simulink model "twin"  (R2018a)
settings: Solver=FixedStepAuto  StartTime=0.0  StopTime=3  FixedStep=0.01  RelTol=1e-3
values from neighbouring files (symbols this model uses):
  B = [-0.5     0       0.5     0 ... (first row only)    [DP_LPCA_based_prio.m]    (also in DPscaled_LPCA_based_prio.m; DPscaled_LPCA_based_prio_by_m1.m; SHC09.m = I \ [-l1, -l1*cos(d),  l1*cos(d),  l1,  l1*cos(d), -l1*cos(d; SHW09_vtol.m = zeros(3, 8))
  plim = [umin umax]    [derivative_DF.m]    (also in difference.m; quad.m; quad_tau.m; restoring_2d.m)
undefined symbols (not defined in the file or in its folder): a_c, a_t, Am, com_c, com_t_dca, com_t_inv, com_t_wls, p_limits, select_test, sigbuilder_block, v_limits
libraries: simulink x4, qcatlib x3, aerolibactuator x3
settings Model: Creator=mengc  LastModifiedBy=Ducted Fan

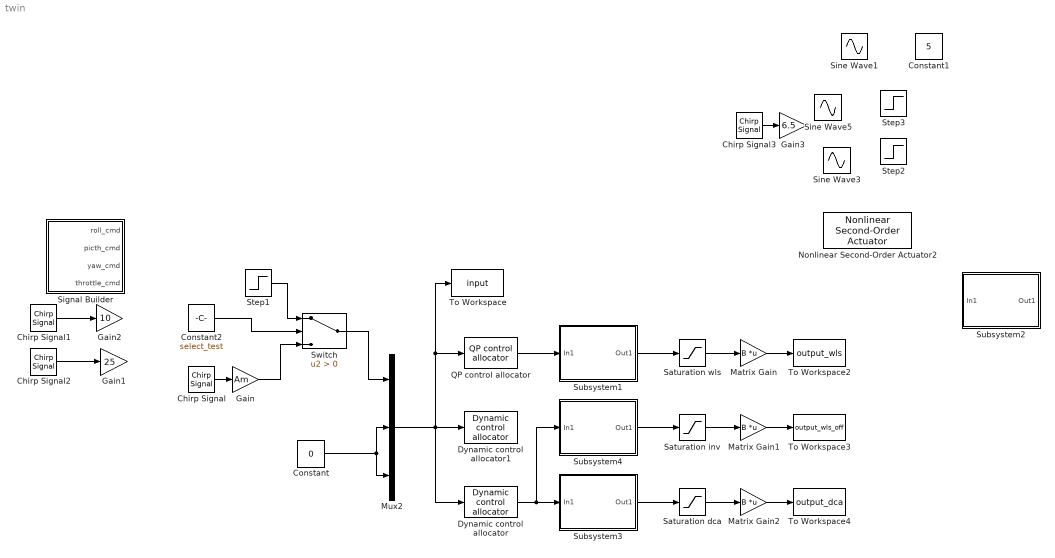
== system twin ==
  Chirp Signal : simulink/Sources/Chirp Signal  f1=lf  T=3  f2=hf
  Chirp Signal1 : simulink/Sources/Chirp Signal  f1=1  T=2  f2=5
  Chirp Signal2 : simulink/Sources/Chirp Signal  f1=1  T=2  f2=5
  Chirp Signal3 : simulink/Sources/Chirp Signal  f1=2  T=2  f2=6
  Constant : Constant  Value=0  SampleTime=0.01
  Constant1 : Constant  Value=5  SampleTime=0.01
  Constant2 : Constant  Value=select_test  SampleTime=0.01
  Dynamic control allocator : qcatlib/Dynamic control allocator  B=B  plim=plim  rlim=rlim  T=0.01  Wv=eye(3)  W1=dca_W1  W2=dca_W2  S=S
      settings: SourceProductName=QP Control Allocation Toolbox
  Dynamic control allocator1 : qcatlib/Dynamic control allocator  B=B  plim=plim  rlim=rlim  T=0.01  Wv=eye(3)  W1=eye(9)  W2=zeros(9,9)  S=S
      settings: SourceProductName=QP Control Allocation Toolbox
  Gain : Gain  Gain=Am
  Gain1 : Gain  Gain=25
  Gain2 : Gain  Gain=10
  Gain3 : Gain  Gain=6.5
  Matrix Gain : Gain  Gain=B  Multiplication=Matrix(K*u)  SaturateOnIntegerOverflow=on  OutDataTypeStr=Inherit: Same as input  ParamDataTypeStr=Inherit: Same as input
  Matrix Gain1 : Gain  Gain=B  Multiplication=Matrix(K*u)  SaturateOnIntegerOverflow=on  OutDataTypeStr=Inherit: Same as input  ParamDataTypeStr=Inherit: Same as input
  Matrix Gain2 : Gain  Gain=B  Multiplication=Matrix(K*u)  SaturateOnIntegerOverflow=on  OutDataTypeStr=Inherit: Same as input  ParamDataTypeStr=Inherit: Same as input
  Mux2 : Mux  Inputs=3
  Nonlinear Second-Order Actuator2 : aerolibactuator/Nonlinear Second-Order Actuator  wn_fin=200  z_fin=0.7  fin_max=umax  fin_min=umin  fin_maxrate=vmax  fin_act_0=zeros(9,1)  fin_act_vel=zeros(9,1)
      settings: SourceProductName=Aerospace Blockset  SourceProductBaseCode=AE
  QP control allocator : qcatlib/QP control allocator  B=B  plim=plim  rlim=rlim  T=0.01  Wv=eye(3)  Wu=eye(9)  ud=zeros(9,1)  alg=WLS  imax=100  gam=1e6  tol=1e-4
      settings: SourceProductName=QP Control Allocation Toolbox
  Saturation dca : Saturate  UpperLimit=plim(:,2)  LowerLimit=plim(:,1)
  Saturation inv : Saturate  UpperLimit=plim(:,2)  LowerLimit=plim(:,1)
  Saturation wls : Saturate  UpperLimit=plim(:,2)  LowerLimit=plim(:,1)
  Signal Builder : Subsystem  Tag=STV Subsys  LoadFcn=sigbuilder_block('load');  StartFcn=sigbuilder_block('start');  StopFcn=sigbuilder_block('stop');  ClipboardFcn=sigbuilder_block('clipboard');  mask(Sigbuilder block){tuvar=[0:10]}
      mask help: Simulink:masks:SigbuilderBlock_MD
      mask init:
      | if ~strcmp(get_param(bdroot(gcbh),'SimulationStatus'),'stopped') tuvar = sigbuilder_block('maskInit'); end
      settings: CopyFcn=sigbuilder_block('copy');  DeleteFcn=sigbuilder_block('delete');  ModelCloseFcn=sigbuilder_block('modelClose');  PreSaveFcn=sigbuilder_block('preSave');  PauseFcn=sigbuilder_block('pause');  ContinueFcn=sigbuilder_block('continue');  NameChangeFcn=sigbuilder_block('namechange');  OpenFcn=sigbuilder_block('open',[42.75 46.5 943.5 423.75 ]);  CloseFcn=sigbuilder_block('close');
      mask Display: plot(0, 0, 100, 100,[2, 2, 32, 32, 2], [68, 8, 8, 68, 68],[32, 2], [38, 38], [32, 19, 2],[53, 60, 44], [32, 17, 17, 2],[16, 16, 31, 31]);txt = getActiveGroup(gcbh);text(2, 100, txt,'verticalAlignment', 'top');
  Sine Wave1 : Sin  Amplitude=12  Frequency=4*pi/2  Phase=pi/2  SampleTime=0.01
  Sine Wave3 : Sin  Amplitude=15  Frequency=4*pi/2  Phase=pi/2  SampleTime=0.01
  Sine Wave5 : Sin  Amplitude=5  Frequency=4*pi/2  SampleTime=0.01
  Step1 : Step  Time=0.2  After=6  SampleTime=0.01
  Step2 : Step  Time=0.5  After=3  SampleTime=0.01
  Step3 : Step  Time=0.5  After=3  SampleTime=0.01
  Subsystem1 : Subsystem
  Subsystem2 : Subsystem
  Subsystem3 : Subsystem
  Subsystem4 : Subsystem
  Switch : Switch  Criteria=u2 > Threshold
  To Workspace : ToWorkspace  VariableName=input  SaveFormat=Timeseries  SampleTime=-1
  To Workspace2 : ToWorkspace  VariableName=output_wls  SaveFormat=Timeseries  SampleTime=-1
  To Workspace3 : ToWorkspace  VariableName=output_wls_off  SaveFormat=Timeseries  SampleTime=-1
  To Workspace4 : ToWorkspace  VariableName=output_dca  SaveFormat=Timeseries  SampleTime=-1
  wires:
  Mux2/1 -> Dynamic control allocator1/1, To Workspace/1, QP control allocator/1, Dynamic control allocator/1
  Matrix Gain/1 -> To Workspace2/1
  Matrix Gain2/1 -> To Workspace4/1
  Dynamic control allocator/1 -> Subsystem3/1(In1), Subsystem4/1(In1)
  Matrix Gain1/1 -> To Workspace3/1
  Subsystem3/1(Out1) -> Saturation dca/1
  Subsystem4/1(Out1) -> Saturation inv/1
  Subsystem1/1(Out1) -> Saturation wls/1
  QP control allocator/1 -> Subsystem1/1(In1)
  Saturation wls/1 -> Matrix Gain/1
  Saturation inv/1 -> Matrix Gain1/1
  Saturation dca/1 -> Matrix Gain2/1
  Chirp Signal2/1 -> Gain1/1
  Chirp Signal1/1 -> Gain2/1
  Chirp Signal/1 -> Gain/1
  Chirp Signal3/1 -> Gain3/1
  Constant/1 -> Mux2/3, Mux2/2
  Step1/1 -> Switch/1
  Gain/1 -> Switch/3
  Constant2/1 -> Switch/2
  Switch/1 -> Mux2/1

== system twin/Signal Builder ==
  Demux : Demux  Tag=STV Demux
  FromWs : FromWorkspace  Tag=STV FromWs  VariableName=tuvar  SampleTime=0
      SigBuilderData=|
      | common.afterFinalStr = 'Extrapolate'
      | common.sampleTime = 0
      | dataSet.timeRange = [0 100]
      | dataSet.name = 'Group 1'
      | sbobj.Groups.Name = 'Group 1'
      | sbobj.Groups.Signals(1).Name = 'roll_cmd'
      | sbobj.Groups.Signals(1).XData = [0 0.5 0.5 100]
      | sbobj.Groups.Signals(1).YData = [0 0 5 10]
      | sbobj.Groups.Signals(2).Name = 'picth_cmd'
      | sbobj.Groups.Signals(2).XData = [0 30 30 100]
      | sbobj.Groups.Signals(2).YData = [-0.0045 -0.0045 0.3 0.3]
      | sbobj.Groups.Signals(3).Name = 'yaw_cmd'
      | sbobj.Groups.Signals(3).XData = [0 30 30 100]
      | sbobj.Groups.Signals(3).YData = [0.0779 0.0779 0.2 0.2]
      | sbobj.Groups.Signals(4).Name = 'throttle_cmd'
      | sbobj.Groups.Signals(4).XData = [0 100]
      | sbobj.Groups.Signals(4).YData = [0 0]
      | sbobj.Groups.TimeRange = [0 100]
  roll_cmd : Outport  Tag=STV Outport
  picth_cmd : Outport  Tag=STV Outport  Port=2
  yaw_cmd : Outport  Tag=STV Outport  Port=3
  throttle_cmd : Outport  Tag=STV Outport  Port=4
  wires:
  Demux/1 -> roll_cmd/1
  FromWs/1 -> Demux/1
  Demux/2 -> picth_cmd/1
  Demux/3 -> yaw_cmd/1
  Demux/4 -> throttle_cmd/1

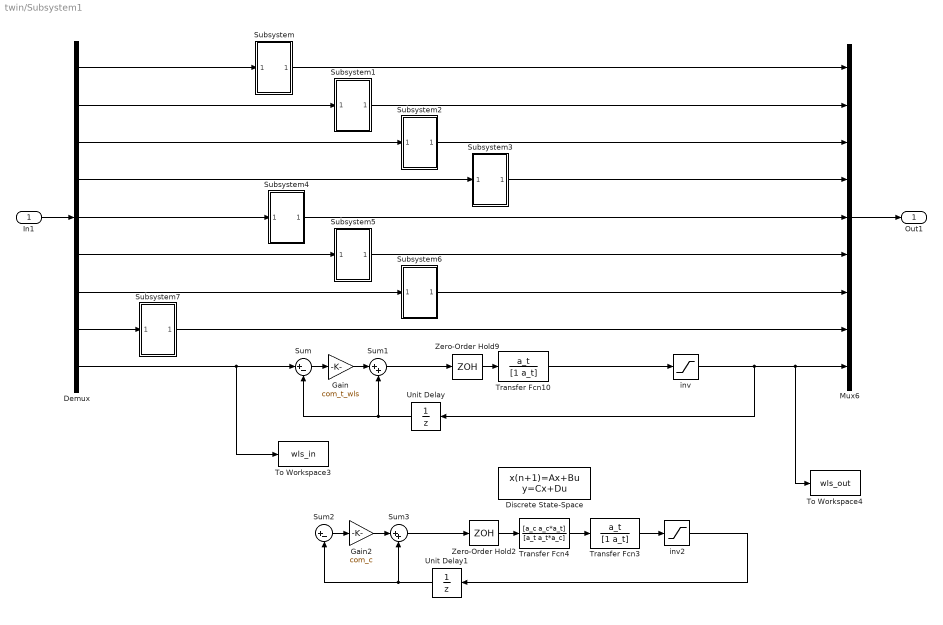
== system twin/Subsystem1 ==
  In1 : Inport
  Demux : Demux  Outputs=9
  Discrete State-Space : DiscreteStateSpace  A=exp(-0.01*a_t)  B=1-exp(-0.01*a_t)  D=0  SampleTime=-1
  Gain : Gain  Gain=com_t_wls
  Gain2 : Gain  Gain=com_c
  Mux6 : Mux  Inputs=9
  Subsystem : Subsystem
  Subsystem1 : Subsystem
  Subsystem2 : Subsystem
  Subsystem3 : Subsystem
  Subsystem4 : Subsystem
  Subsystem5 : Subsystem
  Subsystem6 : Subsystem
  Subsystem7 : Subsystem
  Sum : Sum  Inputs=|+-
  Sum1 : Sum  Inputs=|++
  Sum2 : Sum  Inputs=|+-
  Sum3 : Sum  Inputs=|++
  To Workspace3 : ToWorkspace  VariableName=wls_in  SaveFormat=Timeseries  SampleTime=-1
  To Workspace4 : ToWorkspace  VariableName=wls_out  SaveFormat=Timeseries  SampleTime=-1
  Transfer Fcn10 : TransferFcn  Numerator=a_t  Denominator=[1 a_t]
  Transfer Fcn3 : TransferFcn  Numerator=a_t  Denominator=[1 a_t]
  Transfer Fcn4 : TransferFcn  Numerator=[a_c a_c*a_t]  Denominator=[a_t a_t*a_c]
  Unit Delay : UnitDelay  SampleTime=-1
  Unit Delay1 : UnitDelay  SampleTime=-1
  Zero-Order Hold2 : ZeroOrderHold  SampleTime=-1
  Zero-Order Hold9 : ZeroOrderHold  SampleTime=-1
  inv : Saturate  UpperLimit=p_limits(2)  LowerLimit=-p_limits(2)
  inv2 : Saturate  UpperLimit=p_limits(2)  LowerLimit=-p_limits(2)
  Out1 : Outport
  wires:
  In1/1 -> Demux/1
  Mux6/1 -> Out1/1
  Gain/1 -> Sum1/1
  Zero-Order Hold9/1 -> Transfer Fcn10/1
  Unit Delay/1 -> Sum/2, Sum1/2
  Sum/1 -> Gain/1
  Sum1/1 -> Zero-Order Hold9/1
  Demux/1 -> Subsystem/1(In1)
  Subsystem/1(Out1) -> Mux6/1
  Demux/2 -> Subsystem1/1(In1)
  Subsystem1/1(Out1) -> Mux6/2
  Demux/3 -> Subsystem2/1(In1)
  Subsystem2/1(Out1) -> Mux6/3
  Demux/4 -> Subsystem3/1(In1)
  Subsystem3/1(Out1) -> Mux6/4
  Demux/5 -> Subsystem4/1(In1)
  Subsystem4/1(Out1) -> Mux6/5
  Demux/6 -> Subsystem5/1(In1)
  Subsystem5/1(Out1) -> Mux6/6
  Demux/7 -> Subsystem6/1(In1)
  Subsystem6/1(Out1) -> Mux6/7
  Subsystem7/1(Out1) -> Mux6/8
  Demux/8 -> Subsystem7/1(In1)
  inv/1 -> To Workspace4/1, Mux6/9, Unit Delay/1
  Gain2/1 -> Sum3/1
  Sum2/1 -> Gain2/1
  Unit Delay1/1 -> Sum2/2, Sum3/2
  Transfer Fcn4/1 -> Transfer Fcn3/1
  Transfer Fcn3/1 -> inv2/1
  Zero-Order Hold2/1 -> Transfer Fcn4/1
  inv2/1 -> Unit Delay1/1
  Sum3/1 -> Zero-Order Hold2/1
  Transfer Fcn10/1 -> inv/1
  Demux/9 -> To Workspace3/1, Sum/1

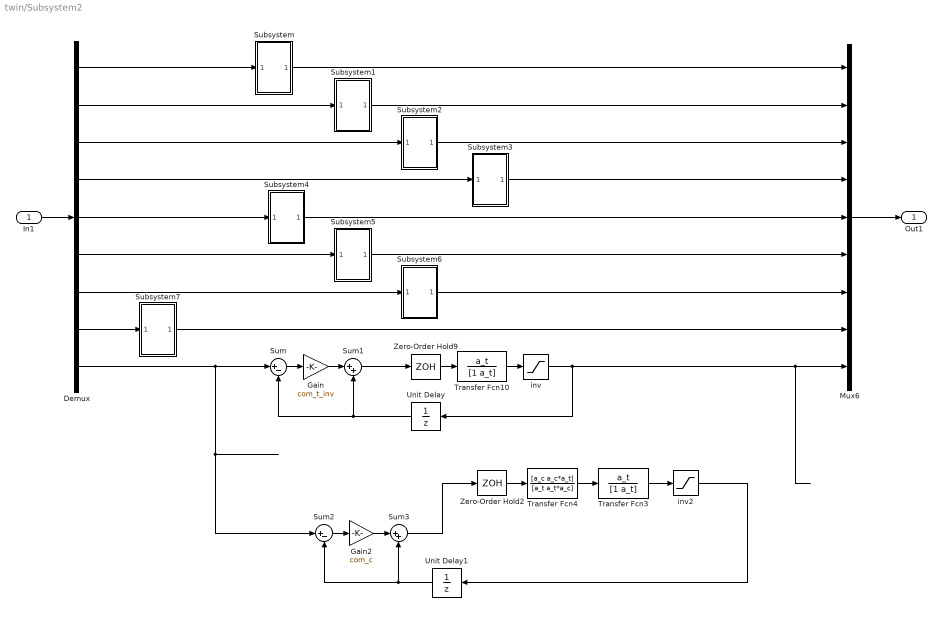
== system twin/Subsystem2 ==
  In1 : Inport
  Demux : Demux  Outputs=9
  Gain : Gain  Gain=com_t_inv
  Gain2 : Gain  Gain=com_c
  Mux6 : Mux  Inputs=9
  Subsystem : Subsystem
  Subsystem1 : Subsystem
  Subsystem2 : Subsystem
  Subsystem3 : Subsystem
  Subsystem4 : Subsystem
  Subsystem5 : Subsystem
  Subsystem6 : Subsystem
  Subsystem7 : Subsystem
  Sum : Sum  Inputs=|+-
  Sum1 : Sum  Inputs=|++
  Sum2 : Sum  Inputs=|+-
  Sum3 : Sum  Inputs=|++
  Transfer Fcn10 : TransferFcn  Numerator=a_t  Denominator=[1 a_t]
  Transfer Fcn3 : TransferFcn  Numerator=a_t  Denominator=[1 a_t]
  Transfer Fcn4 : TransferFcn  Numerator=[a_c a_c*a_t]  Denominator=[a_t a_t*a_c]
  Unit Delay : UnitDelay  SampleTime=-1
  Unit Delay1 : UnitDelay  SampleTime=-1
  Zero-Order Hold2 : ZeroOrderHold  SampleTime=-1
  Zero-Order Hold9 : ZeroOrderHold  SampleTime=-1
  inv : Saturate  UpperLimit=p_limits(2)  LowerLimit=-p_limits(2)
  inv2 : Saturate  UpperLimit=p_limits(2)  LowerLimit=-p_limits(2)
  Out1 : Outport
  wires:
  In1/1 -> Demux/1
  Mux6/1 -> Out1/1
  Transfer Fcn10/1 -> inv/1
  Gain/1 -> Sum1/1
  Zero-Order Hold9/1 -> Transfer Fcn10/1
  Unit Delay/1 -> Sum/2, Sum1/2
  Sum/1 -> Gain/1
  Demux/1 -> Subsystem/1(In1)
  Subsystem/1(Out1) -> Mux6/1
  Demux/2 -> Subsystem1/1(In1)
  Subsystem1/1(Out1) -> Mux6/2
  Demux/3 -> Subsystem2/1(In1)
  Subsystem2/1(Out1) -> Mux6/3
  Demux/4 -> Subsystem3/1(In1)
  Subsystem3/1(Out1) -> Mux6/4
  Demux/5 -> Subsystem4/1(In1)
  Subsystem4/1(Out1) -> Mux6/5
  Demux/6 -> Subsystem5/1(In1)
  Subsystem5/1(Out1) -> Mux6/6
  Demux/7 -> Subsystem6/1(In1)
  Subsystem6/1(Out1) -> Mux6/7
  Subsystem7/1(Out1) -> Mux6/8
  Demux/8 -> Subsystem7/1(In1)
  inv/1 -> Mux6/9, Unit Delay/1
  Gain2/1 -> Sum3/1
  Sum2/1 -> Gain2/1
  Unit Delay1/1 -> Sum2/2, Sum3/2
  Transfer Fcn4/1 -> Transfer Fcn3/1
  Transfer Fcn3/1 -> inv2/1
  Zero-Order Hold2/1 -> Transfer Fcn4/1
  inv2/1 -> Unit Delay1/1
  Sum3/1 -> Zero-Order Hold2/1
  Demux/9 -> Sum/1, Sum2/1
  Sum1/1 -> Zero-Order Hold9/1

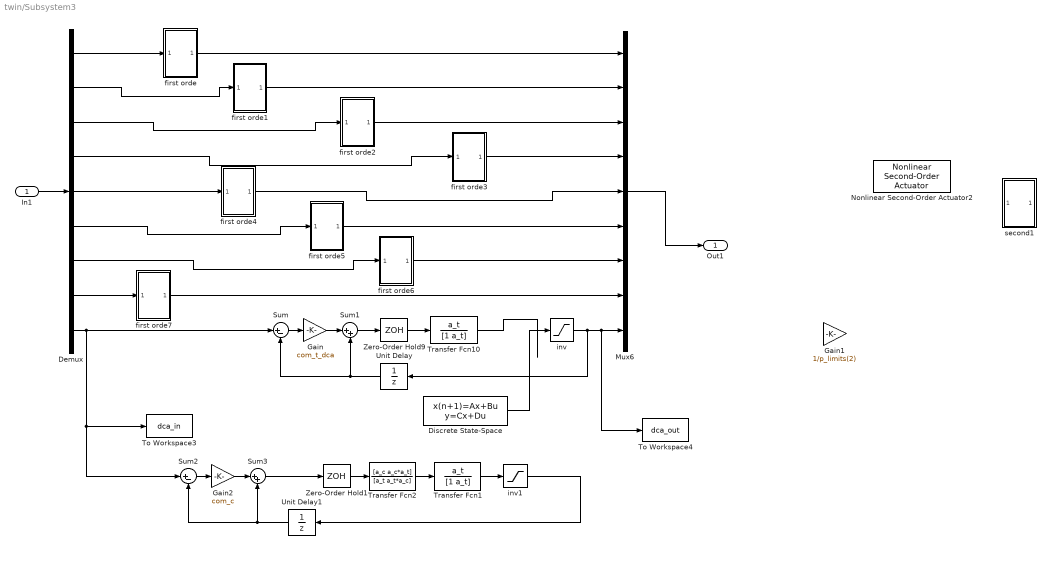
== system twin/Subsystem3 ==
  In1 : Inport
  Demux : Demux  Outputs=9
  Discrete State-Space : DiscreteStateSpace  A=exp(-0.01*a_t)  B=1-exp(-0.01*a_t)  D=0  SampleTime=-1
  Gain : Gain  Gain=com_t_dca
  Gain1 : Gain  Gain=1/p_limits(2)
  Gain2 : Gain  Gain=com_c
  Mux6 : Mux  Inputs=9
  Nonlinear Second-Order Actuator2 : aerolibactuator/Nonlinear Second-Order Actuator  wn_fin=200  z_fin=0.7  fin_max=(p_limits(2))*pi/180  fin_min=(-p_limits(2))*pi/180  fin_maxrate=v_limits(2)  fin_act_0=0  fin_act_vel=0
      settings: SourceProductName=Aerospace Blockset  SourceProductBaseCode=AE
  Sum : Sum  Inputs=|+-
  Sum1 : Sum  Inputs=|++
  Sum2 : Sum  Inputs=|+-
  Sum3 : Sum  Inputs=|++
  To Workspace3 : ToWorkspace  VariableName=dca_in  SaveFormat=Timeseries  SampleTime=-1
  To Workspace4 : ToWorkspace  VariableName=dca_out  SaveFormat=Timeseries  SampleTime=-1
  Transfer Fcn1 : TransferFcn  Numerator=a_t  Denominator=[1 a_t]
  Transfer Fcn10 : TransferFcn  Numerator=a_t  Denominator=[1 a_t]
  Transfer Fcn2 : TransferFcn  Numerator=[a_c a_c*a_t]  Denominator=[a_t a_t*a_c]
  Unit Delay : UnitDelay  SampleTime=-1
  Unit Delay1 : UnitDelay  SampleTime=-1
  Zero-Order Hold1 : ZeroOrderHold  SampleTime=-1
  Zero-Order Hold9 : ZeroOrderHold  SampleTime=-1
  first orde : Subsystem
  first orde1 : Subsystem
  first orde2 : Subsystem
  first orde3 : Subsystem
  first orde4 : Subsystem
  first orde5 : Subsystem
  first orde6 : Subsystem
  first orde7 : Subsystem
  inv : Saturate  UpperLimit=p_limits(2)  LowerLimit=-p_limits(2)
  inv1 : Saturate  UpperLimit=p_limits(2)  LowerLimit=-p_limits(2)
  second1 : Subsystem
  Out1 : Outport
  wires:
  In1/1 -> Demux/1
  Mux6/1 -> Out1/1
  Gain/1 -> Sum1/1
  Unit Delay/1 -> Sum/2, Sum1/2
  Sum/1 -> Gain/1
  Sum1/1 -> Zero-Order Hold9/1
  Demux/1 -> first orde/1(In1)
  first orde/1(Out1) -> Mux6/1
  Demux/2 -> first orde1/1(In1)
  first orde1/1(Out1) -> Mux6/2
  Demux/3 -> first orde2/1(In1)
  first orde2/1(Out1) -> Mux6/3
  Demux/4 -> first orde3/1(In1)
  first orde3/1(Out1) -> Mux6/4
  Demux/5 -> first orde4/1(In1)
  first orde4/1(Out1) -> Mux6/5
  Demux/6 -> first orde5/1(In1)
  first orde5/1(Out1) -> Mux6/6
  Demux/7 -> first orde6/1(In1)
  first orde6/1(Out1) -> Mux6/7
  first orde7/1(Out1) -> Mux6/8
  Demux/8 -> first orde7/1(In1)
  Transfer Fcn10/1 -> inv/1
  inv/1 -> To Workspace4/1, Mux6/9, Unit Delay/1
  Transfer Fcn1/1 -> inv1/1
  Zero-Order Hold1/1 -> Transfer Fcn2/1
  Transfer Fcn2/1 -> Transfer Fcn1/1
  inv1/1 -> Unit Delay1/1
  Sum3/1 -> Zero-Order Hold1/1
  Unit Delay1/1 -> Sum2/2, Sum3/2
  Sum2/1 -> Gain2/1
  Gain2/1 -> Sum3/1
  Demux/9 -> Sum2/1, To Workspace3/1, Sum/1
  Discrete State-Space/1 -> ?
  Zero-Order Hold9/1 -> Transfer Fcn10/1

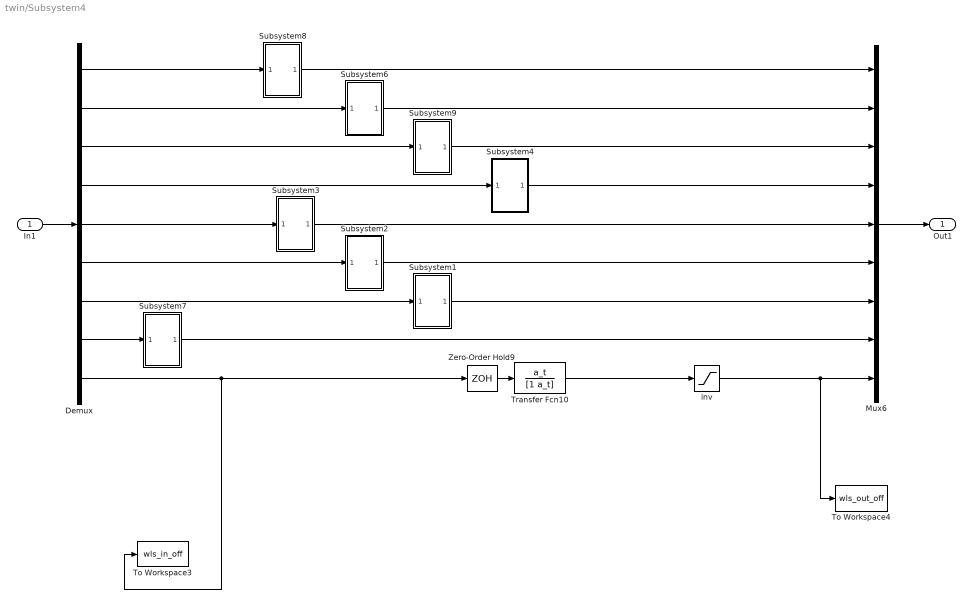
== system twin/Subsystem4 ==
  In1 : Inport
  Demux : Demux  Outputs=9
  Mux6 : Mux  Inputs=9
  Subsystem1 : Subsystem
  Subsystem2 : Subsystem
  Subsystem3 : Subsystem
  Subsystem4 : Subsystem
  Subsystem6 : Subsystem
  Subsystem7 : Subsystem
  Subsystem8 : Subsystem
  Subsystem9 : Subsystem
  To Workspace3 : ToWorkspace  VariableName=wls_in_off  SaveFormat=Timeseries  SampleTime=-1
  To Workspace4 : ToWorkspace  VariableName=wls_out_off  SaveFormat=Timeseries  SampleTime=-1
  Transfer Fcn10 : TransferFcn  Numerator=a_t  Denominator=[1 a_t]
  Zero-Order Hold9 : ZeroOrderHold  SampleTime=-1
  inv : Saturate  UpperLimit=p_limits(2)  LowerLimit=-p_limits(2)
  Out1 : Outport
  wires:
  In1/1 -> Demux/1
  Mux6/1 -> Out1/1
  Zero-Order Hold9/1 -> Transfer Fcn10/1
  Demux/1 -> Subsystem8/1(In1)
  Subsystem8/1(Out1) -> Mux6/1
  Demux/2 -> Subsystem6/1(In1)
  Subsystem6/1(Out1) -> Mux6/2
  Demux/3 -> Subsystem9/1(In1)
  Subsystem9/1(Out1) -> Mux6/3
  Demux/4 -> Subsystem4/1(In1)
  Subsystem4/1(Out1) -> Mux6/4
  Demux/5 -> Subsystem3/1(In1)
  Subsystem3/1(Out1) -> Mux6/5
  Demux/6 -> Subsystem2/1(In1)
  Subsystem2/1(Out1) -> Mux6/6
  Demux/7 -> Subsystem1/1(In1)
  Subsystem1/1(Out1) -> Mux6/7
  Subsystem7/1(Out1) -> Mux6/8
  Demux/8 -> Subsystem7/1(In1)
  inv/1 -> To Workspace4/1, Mux6/9
  Demux/9 -> Zero-Order Hold9/1, To Workspace3/1
  Transfer Fcn10/1 -> inv/1

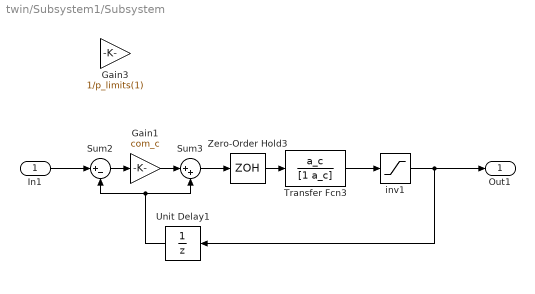
== system twin/Subsystem1/Subsystem ==
  In1 : Inport
  Gain1 : Gain  Gain=com_c
  Gain3 : Gain  Gain=1/p_limits(1)
  Sum2 : Sum  Inputs=|+-
  Sum3 : Sum  Inputs=|++
  Transfer Fcn3 : TransferFcn  Numerator=a_c  Denominator=[1 a_c]
  Unit Delay1 : UnitDelay  SampleTime=-1
  Zero-Order Hold3 : ZeroOrderHold  SampleTime=-1
  inv1 : Saturate  UpperLimit=p_limits(1)  LowerLimit=-p_limits(1)
  Out1 : Outport
  wires:
  Transfer Fcn3/1 -> inv1/1
  Gain1/1 -> Sum3/1
  Unit Delay1/1 -> Sum2/2, Sum3/2
  Sum2/1 -> Gain1/1
  Zero-Order Hold3/1 -> Transfer Fcn3/1
  Sum3/1 -> Zero-Order Hold3/1
  inv1/1 -> Unit Delay1/1, Out1/1
  In1/1 -> Sum2/1

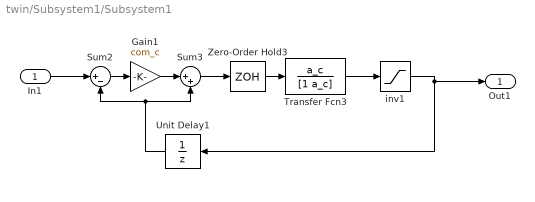
== system twin/Subsystem1/Subsystem1 ==
  In1 : Inport
  Gain1 : Gain  Gain=com_c
  Sum2 : Sum  Inputs=|+-
  Sum3 : Sum  Inputs=|++
  Transfer Fcn3 : TransferFcn  Numerator=a_c  Denominator=[1 a_c]
  Unit Delay1 : UnitDelay  SampleTime=-1
  Zero-Order Hold3 : ZeroOrderHold  SampleTime=-1
  inv1 : Saturate  UpperLimit=p_limits(1)  LowerLimit=-p_limits(1)
  Out1 : Outport
  wires:
  Transfer Fcn3/1 -> inv1/1
  Gain1/1 -> Sum3/1
  inv1/1 -> Unit Delay1/1, Out1/1
  In1/1 -> Sum2/1
  Unit Delay1/1 -> Sum2/2, Sum3/2
  Sum2/1 -> Gain1/1
  Zero-Order Hold3/1 -> Transfer Fcn3/1
  Sum3/1 -> Zero-Order Hold3/1

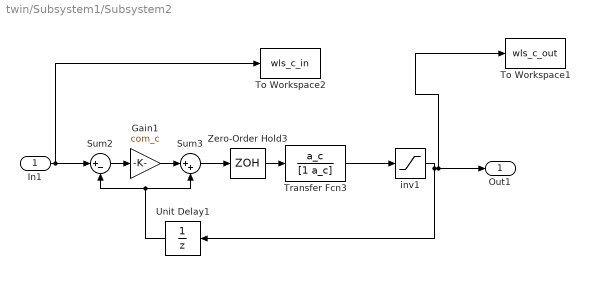
== system twin/Subsystem1/Subsystem2 ==
  In1 : Inport
  Gain1 : Gain  Gain=com_c
  Sum2 : Sum  Inputs=|+-
  Sum3 : Sum  Inputs=|++
  To Workspace1 : ToWorkspace  VariableName=wls_c_out  SaveFormat=Timeseries  SampleTime=-1
  To Workspace2 : ToWorkspace  VariableName=wls_c_in  SaveFormat=Timeseries  SampleTime=-1
  Transfer Fcn3 : TransferFcn  Numerator=a_c  Denominator=[1 a_c]
  Unit Delay1 : UnitDelay  SampleTime=-1
  Zero-Order Hold3 : ZeroOrderHold  SampleTime=-1
  inv1 : Saturate  UpperLimit=p_limits(1)  LowerLimit=-p_limits(1)
  Out1 : Outport
  wires:
  Gain1/1 -> Sum3/1
  Unit Delay1/1 -> Sum2/2, Sum3/2
  Sum2/1 -> Gain1/1
  Zero-Order Hold3/1 -> Transfer Fcn3/1
  Sum3/1 -> Zero-Order Hold3/1
  In1/1 -> To Workspace2/1, Sum2/1
  inv1/1 -> Unit Delay1/1, To Workspace1/1, Out1/1
  Transfer Fcn3/1 -> inv1/1

== system twin/Subsystem1/Subsystem3 ==
  In1 : Inport
  Gain1 : Gain  Gain=com_c
  Sum2 : Sum  Inputs=|+-
  Sum3 : Sum  Inputs=|++
  Transfer Fcn3 : TransferFcn  Numerator=a_c  Denominator=[1 a_c]
  Unit Delay1 : UnitDelay  SampleTime=-1
  Zero-Order Hold3 : ZeroOrderHold  SampleTime=-1
  inv1 : Saturate  UpperLimit=p_limits(1)  LowerLimit=-p_limits(1)
  Out1 : Outport
  wires:
  Transfer Fcn3/1 -> inv1/1
  Gain1/1 -> Sum3/1
  inv1/1 -> Unit Delay1/1, Out1/1
  In1/1 -> Sum2/1
  Unit Delay1/1 -> Sum2/2, Sum3/2
  Sum2/1 -> Gain1/1
  Zero-Order Hold3/1 -> Transfer Fcn3/1
  Sum3/1 -> Zero-Order Hold3/1

== system twin/Subsystem1/Subsystem4 ==
  In1 : Inport
  Gain1 : Gain  Gain=com_c
  Sum2 : Sum  Inputs=|+-
  Sum3 : Sum  Inputs=|++
  Transfer Fcn3 : TransferFcn  Numerator=a_c  Denominator=[1 a_c]
  Unit Delay1 : UnitDelay  SampleTime=-1
  Zero-Order Hold3 : ZeroOrderHold  SampleTime=-1
  inv1 : Saturate  UpperLimit=p_limits(1)  LowerLimit=-p_limits(1)
  Out1 : Outport
  wires:
  Transfer Fcn3/1 -> inv1/1
  Gain1/1 -> Sum3/1
  inv1/1 -> Unit Delay1/1, Out1/1
  In1/1 -> Sum2/1
  Unit Delay1/1 -> Sum2/2, Sum3/2
  Sum2/1 -> Gain1/1
  Zero-Order Hold3/1 -> Transfer Fcn3/1
  Sum3/1 -> Zero-Order Hold3/1

== system twin/Subsystem1/Subsystem5 ==
  In1 : Inport
  Gain1 : Gain  Gain=com_c
  Sum2 : Sum  Inputs=|+-
  Sum3 : Sum  Inputs=|++
  Transfer Fcn3 : TransferFcn  Numerator=a_c  Denominator=[1 a_c]
  Unit Delay1 : UnitDelay  SampleTime=-1
  Zero-Order Hold3 : ZeroOrderHold  SampleTime=-1
  inv1 : Saturate  UpperLimit=p_limits(1)  LowerLimit=-p_limits(1)
  Out1 : Outport
  wires:
  Transfer Fcn3/1 -> inv1/1
  Gain1/1 -> Sum3/1
  inv1/1 -> Unit Delay1/1, Out1/1
  In1/1 -> Sum2/1
  Unit Delay1/1 -> Sum2/2, Sum3/2
  Sum2/1 -> Gain1/1
  Zero-Order Hold3/1 -> Transfer Fcn3/1
  Sum3/1 -> Zero-Order Hold3/1

== system twin/Subsystem1/Subsystem6 ==
  In1 : Inport
  Gain1 : Gain  Gain=com_c
  Sum2 : Sum  Inputs=|+-
  Sum3 : Sum  Inputs=|++
  Transfer Fcn3 : TransferFcn  Numerator=a_c  Denominator=[1 a_c]
  Unit Delay1 : UnitDelay  SampleTime=-1
  Zero-Order Hold3 : ZeroOrderHold  SampleTime=-1
  inv1 : Saturate  UpperLimit=p_limits(1)  LowerLimit=-p_limits(1)
  Out1 : Outport
  wires:
  Transfer Fcn3/1 -> inv1/1
  Gain1/1 -> Sum3/1
  inv1/1 -> Unit Delay1/1, Out1/1
  In1/1 -> Sum2/1
  Unit Delay1/1 -> Sum2/2, Sum3/2
  Sum2/1 -> Gain1/1
  Zero-Order Hold3/1 -> Transfer Fcn3/1
  Sum3/1 -> Zero-Order Hold3/1

== system twin/Subsystem1/Subsystem7 ==
  In1 : Inport
  Gain1 : Gain  Gain=com_c
  Sum2 : Sum  Inputs=|+-
  Sum3 : Sum  Inputs=|++
  Transfer Fcn3 : TransferFcn  Numerator=a_c  Denominator=[1 a_c]
  Unit Delay1 : UnitDelay  SampleTime=-1
  Zero-Order Hold3 : ZeroOrderHold  SampleTime=-1
  inv1 : Saturate  UpperLimit=p_limits(1)  LowerLimit=-p_limits(1)
  Out1 : Outport
  wires:
  Transfer Fcn3/1 -> inv1/1
  Gain1/1 -> Sum3/1
  inv1/1 -> Unit Delay1/1, Out1/1
  In1/1 -> Sum2/1
  Unit Delay1/1 -> Sum2/2, Sum3/2
  Sum2/1 -> Gain1/1
  Zero-Order Hold3/1 -> Transfer Fcn3/1
  Sum3/1 -> Zero-Order Hold3/1

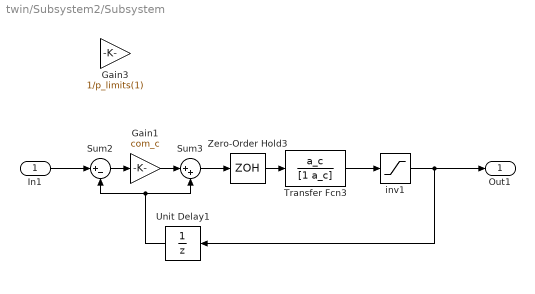
== system twin/Subsystem2/Subsystem ==
  In1 : Inport
  Gain1 : Gain  Gain=com_c
  Gain3 : Gain  Gain=1/p_limits(1)
  Sum2 : Sum  Inputs=|+-
  Sum3 : Sum  Inputs=|++
  Transfer Fcn3 : TransferFcn  Numerator=a_c  Denominator=[1 a_c]
  Unit Delay1 : UnitDelay  SampleTime=-1
  Zero-Order Hold3 : ZeroOrderHold  SampleTime=-1
  inv1 : Saturate  UpperLimit=p_limits(1)  LowerLimit=-p_limits(1)
  Out1 : Outport
  wires:
  Transfer Fcn3/1 -> inv1/1
  Gain1/1 -> Sum3/1
  Unit Delay1/1 -> Sum2/2, Sum3/2
  Sum2/1 -> Gain1/1
  Zero-Order Hold3/1 -> Transfer Fcn3/1
  Sum3/1 -> Zero-Order Hold3/1
  inv1/1 -> Unit Delay1/1, Out1/1
  In1/1 -> Sum2/1

== system twin/Subsystem2/Subsystem1 ==
  In1 : Inport
  Gain1 : Gain  Gain=com_c
  Sum2 : Sum  Inputs=|+-
  Sum3 : Sum  Inputs=|++
  Transfer Fcn3 : TransferFcn  Numerator=a_c  Denominator=[1 a_c]
  Unit Delay1 : UnitDelay  SampleTime=-1
  Zero-Order Hold3 : ZeroOrderHold  SampleTime=-1
  inv1 : Saturate  UpperLimit=p_limits(1)  LowerLimit=-p_limits(1)
  Out1 : Outport
  wires:
  Transfer Fcn3/1 -> inv1/1
  Gain1/1 -> Sum3/1
  inv1/1 -> Unit Delay1/1, Out1/1
  In1/1 -> Sum2/1
  Unit Delay1/1 -> Sum2/2, Sum3/2
  Sum2/1 -> Gain1/1
  Zero-Order Hold3/1 -> Transfer Fcn3/1
  Sum3/1 -> Zero-Order Hold3/1

== system twin/Subsystem2/Subsystem2 ==
  In1 : Inport
  Gain1 : Gain  Gain=com_c
  Sum2 : Sum  Inputs=|+-
  Sum3 : Sum  Inputs=|++
  Transfer Fcn3 : TransferFcn  Numerator=a_c  Denominator=[1 a_c]
  Unit Delay1 : UnitDelay  SampleTime=-1
  Zero-Order Hold3 : ZeroOrderHold  SampleTime=-1
  inv1 : Saturate  UpperLimit=p_limits(1)  LowerLimit=-p_limits(1)
  Out1 : Outport
  wires:
  Transfer Fcn3/1 -> inv1/1
  Gain1/1 -> Sum3/1
  inv1/1 -> Unit Delay1/1, Out1/1
  In1/1 -> Sum2/1
  Unit Delay1/1 -> Sum2/2, Sum3/2
  Sum2/1 -> Gain1/1
  Zero-Order Hold3/1 -> Transfer Fcn3/1
  Sum3/1 -> Zero-Order Hold3/1

== system twin/Subsystem2/Subsystem3 ==
  In1 : Inport
  Gain1 : Gain  Gain=com_c
  Sum2 : Sum  Inputs=|+-
  Sum3 : Sum  Inputs=|++
  Transfer Fcn3 : TransferFcn  Numerator=a_c  Denominator=[1 a_c]
  Unit Delay1 : UnitDelay  SampleTime=-1
  Zero-Order Hold3 : ZeroOrderHold  SampleTime=-1
  inv1 : Saturate  UpperLimit=p_limits(1)  LowerLimit=-p_limits(1)
  Out1 : Outport
  wires:
  Transfer Fcn3/1 -> inv1/1
  Gain1/1 -> Sum3/1
  inv1/1 -> Unit Delay1/1, Out1/1
  In1/1 -> Sum2/1
  Unit Delay1/1 -> Sum2/2, Sum3/2
  Sum2/1 -> Gain1/1
  Zero-Order Hold3/1 -> Transfer Fcn3/1
  Sum3/1 -> Zero-Order Hold3/1

== system twin/Subsystem2/Subsystem4 ==
  In1 : Inport
  Gain1 : Gain  Gain=com_c
  Sum2 : Sum  Inputs=|+-
  Sum3 : Sum  Inputs=|++
  Transfer Fcn3 : TransferFcn  Numerator=a_c  Denominator=[1 a_c]
  Unit Delay1 : UnitDelay  SampleTime=-1
  Zero-Order Hold3 : ZeroOrderHold  SampleTime=-1
  inv1 : Saturate  UpperLimit=p_limits(1)  LowerLimit=-p_limits(1)
  Out1 : Outport
  wires:
  Transfer Fcn3/1 -> inv1/1
  Gain1/1 -> Sum3/1
  inv1/1 -> Unit Delay1/1, Out1/1
  In1/1 -> Sum2/1
  Unit Delay1/1 -> Sum2/2, Sum3/2
  Sum2/1 -> Gain1/1
  Zero-Order Hold3/1 -> Transfer Fcn3/1
  Sum3/1 -> Zero-Order Hold3/1

== system twin/Subsystem2/Subsystem5 ==
  In1 : Inport
  Gain1 : Gain  Gain=com_c
  Sum2 : Sum  Inputs=|+-
  Sum3 : Sum  Inputs=|++
  Transfer Fcn3 : TransferFcn  Numerator=a_c  Denominator=[1 a_c]
  Unit Delay1 : UnitDelay  SampleTime=-1
  Zero-Order Hold3 : ZeroOrderHold  SampleTime=-1
  inv1 : Saturate  UpperLimit=p_limits(1)  LowerLimit=-p_limits(1)
  Out1 : Outport
  wires:
  Transfer Fcn3/1 -> inv1/1
  Gain1/1 -> Sum3/1
  inv1/1 -> Unit Delay1/1, Out1/1
  In1/1 -> Sum2/1
  Unit Delay1/1 -> Sum2/2, Sum3/2
  Sum2/1 -> Gain1/1
  Zero-Order Hold3/1 -> Transfer Fcn3/1
  Sum3/1 -> Zero-Order Hold3/1

== system twin/Subsystem2/Subsystem6 ==
  In1 : Inport
  Gain1 : Gain  Gain=com_c
  Sum2 : Sum  Inputs=|+-
  Sum3 : Sum  Inputs=|++
  Transfer Fcn3 : TransferFcn  Numerator=a_c  Denominator=[1 a_c]
  Unit Delay1 : UnitDelay  SampleTime=-1
  Zero-Order Hold3 : ZeroOrderHold  SampleTime=-1
  inv1 : Saturate  UpperLimit=p_limits(1)  LowerLimit=-p_limits(1)
  Out1 : Outport
  wires:
  Transfer Fcn3/1 -> inv1/1
  Gain1/1 -> Sum3/1
  inv1/1 -> Unit Delay1/1, Out1/1
  In1/1 -> Sum2/1
  Unit Delay1/1 -> Sum2/2, Sum3/2
  Sum2/1 -> Gain1/1
  Zero-Order Hold3/1 -> Transfer Fcn3/1
  Sum3/1 -> Zero-Order Hold3/1

== system twin/Subsystem2/Subsystem7 ==
  In1 : Inport
  Gain1 : Gain  Gain=com_c
  Sum2 : Sum  Inputs=|+-
  Sum3 : Sum  Inputs=|++
  Transfer Fcn3 : TransferFcn  Numerator=a_c  Denominator=[1 a_c]
  Unit Delay1 : UnitDelay  SampleTime=-1
  Zero-Order Hold3 : ZeroOrderHold  SampleTime=-1
  inv1 : Saturate  UpperLimit=p_limits(1)  LowerLimit=-p_limits(1)
  Out1 : Outport
  wires:
  Transfer Fcn3/1 -> inv1/1
  Gain1/1 -> Sum3/1
  inv1/1 -> Unit Delay1/1, Out1/1
  In1/1 -> Sum2/1
  Unit Delay1/1 -> Sum2/2, Sum3/2
  Sum2/1 -> Gain1/1
  Zero-Order Hold3/1 -> Transfer Fcn3/1
  Sum3/1 -> Zero-Order Hold3/1

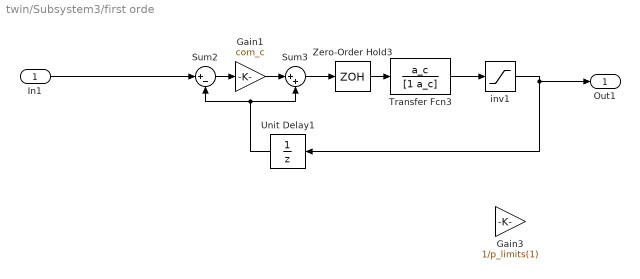
== system twin/Subsystem3/first orde ==
  In1 : Inport
  Gain1 : Gain  Gain=com_c
  Gain3 : Gain  Gain=1/p_limits(1)
  Sum2 : Sum  Inputs=|+-
  Sum3 : Sum  Inputs=|++
  Transfer Fcn3 : TransferFcn  Numerator=a_c  Denominator=[1 a_c]
  Unit Delay1 : UnitDelay  SampleTime=-1
  Zero-Order Hold3 : ZeroOrderHold  SampleTime=-1
  inv1 : Saturate  UpperLimit=p_limits(1)  LowerLimit=-p_limits(1)
  Out1 : Outport
  wires:
  Transfer Fcn3/1 -> inv1/1
  Gain1/1 -> Sum3/1
  Unit Delay1/1 -> Sum2/2, Sum3/2
  Sum2/1 -> Gain1/1
  Zero-Order Hold3/1 -> Transfer Fcn3/1
  Sum3/1 -> Zero-Order Hold3/1
  In1/1 -> Sum2/1
  inv1/1 -> Unit Delay1/1, Out1/1

== system twin/Subsystem3/first orde1 ==
  In1 : Inport
  Gain1 : Gain  Gain=com_c
  Sum2 : Sum  Inputs=|+-
  Sum3 : Sum  Inputs=|++
  Transfer Fcn3 : TransferFcn  Numerator=a_c  Denominator=[1 a_c]
  Unit Delay1 : UnitDelay  SampleTime=-1
  Zero-Order Hold3 : ZeroOrderHold  SampleTime=-1
  inv1 : Saturate  UpperLimit=p_limits(1)  LowerLimit=-p_limits(1)
  Out1 : Outport
  wires:
  Transfer Fcn3/1 -> inv1/1
  Gain1/1 -> Sum3/1
  inv1/1 -> Unit Delay1/1, Out1/1
  In1/1 -> Sum2/1
  Unit Delay1/1 -> Sum2/2, Sum3/2
  Sum2/1 -> Gain1/1
  Zero-Order Hold3/1 -> Transfer Fcn3/1
  Sum3/1 -> Zero-Order Hold3/1

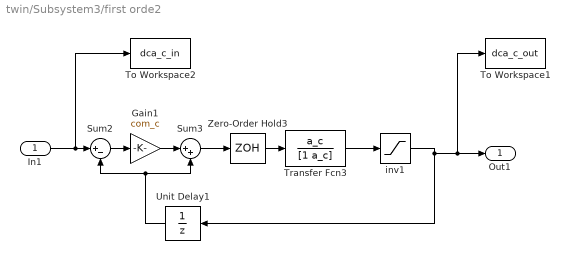
== system twin/Subsystem3/first orde2 ==
  In1 : Inport
  Gain1 : Gain  Gain=com_c
  Sum2 : Sum  Inputs=|+-
  Sum3 : Sum  Inputs=|++
  To Workspace1 : ToWorkspace  VariableName=dca_c_out  SaveFormat=Timeseries  SampleTime=-1
  To Workspace2 : ToWorkspace  VariableName=dca_c_in  SaveFormat=Timeseries  SampleTime=-1
  Transfer Fcn3 : TransferFcn  Numerator=a_c  Denominator=[1 a_c]
  Unit Delay1 : UnitDelay  SampleTime=-1
  Zero-Order Hold3 : ZeroOrderHold  SampleTime=-1
  inv1 : Saturate  UpperLimit=p_limits(1)  LowerLimit=-p_limits(1)
  Out1 : Outport
  wires:
  Transfer Fcn3/1 -> inv1/1
  Gain1/1 -> Sum3/1
  Unit Delay1/1 -> Sum2/2, Sum3/2
  Sum2/1 -> Gain1/1
  Zero-Order Hold3/1 -> Transfer Fcn3/1
  Sum3/1 -> Zero-Order Hold3/1
  inv1/1 -> Unit Delay1/1, To Workspace1/1, Out1/1
  In1/1 -> To Workspace2/1, Sum2/1

== system twin/Subsystem3/first orde3 ==
  In1 : Inport
  Gain1 : Gain  Gain=com_c
  Sum2 : Sum  Inputs=|+-
  Sum3 : Sum  Inputs=|++
  Transfer Fcn3 : TransferFcn  Numerator=a_c  Denominator=[1 a_c]
  Unit Delay1 : UnitDelay  SampleTime=-1
  Zero-Order Hold3 : ZeroOrderHold  SampleTime=-1
  inv1 : Saturate  UpperLimit=p_limits(1)  LowerLimit=-p_limits(1)
  Out1 : Outport
  wires:
  Transfer Fcn3/1 -> inv1/1
  Gain1/1 -> Sum3/1
  inv1/1 -> Unit Delay1/1, Out1/1
  In1/1 -> Sum2/1
  Unit Delay1/1 -> Sum2/2, Sum3/2
  Sum2/1 -> Gain1/1
  Zero-Order Hold3/1 -> Transfer Fcn3/1
  Sum3/1 -> Zero-Order Hold3/1

== system twin/Subsystem3/first orde4 ==
  In1 : Inport
  Gain1 : Gain  Gain=com_c
  Sum2 : Sum  Inputs=|+-
  Sum3 : Sum  Inputs=|++
  Transfer Fcn3 : TransferFcn  Numerator=a_c  Denominator=[1 a_c]
  Unit Delay1 : UnitDelay  SampleTime=-1
  Zero-Order Hold3 : ZeroOrderHold  SampleTime=-1
  inv1 : Saturate  UpperLimit=p_limits(1)  LowerLimit=-p_limits(1)
  Out1 : Outport
  wires:
  Transfer Fcn3/1 -> inv1/1
  Gain1/1 -> Sum3/1
  inv1/1 -> Unit Delay1/1, Out1/1
  In1/1 -> Sum2/1
  Unit Delay1/1 -> Sum2/2, Sum3/2
  Sum2/1 -> Gain1/1
  Zero-Order Hold3/1 -> Transfer Fcn3/1
  Sum3/1 -> Zero-Order Hold3/1

== system twin/Subsystem3/first orde5 ==
  In1 : Inport
  Gain1 : Gain  Gain=com_c
  Sum2 : Sum  Inputs=|+-
  Sum3 : Sum  Inputs=|++
  Transfer Fcn3 : TransferFcn  Numerator=a_c  Denominator=[1 a_c]
  Unit Delay1 : UnitDelay  SampleTime=-1
  Zero-Order Hold3 : ZeroOrderHold  SampleTime=-1
  inv1 : Saturate  UpperLimit=p_limits(1)  LowerLimit=-p_limits(1)
  Out1 : Outport
  wires:
  Transfer Fcn3/1 -> inv1/1
  Gain1/1 -> Sum3/1
  inv1/1 -> Unit Delay1/1, Out1/1
  In1/1 -> Sum2/1
  Unit Delay1/1 -> Sum2/2, Sum3/2
  Sum2/1 -> Gain1/1
  Zero-Order Hold3/1 -> Transfer Fcn3/1
  Sum3/1 -> Zero-Order Hold3/1

== system twin/Subsystem3/first orde6 ==
  In1 : Inport
  Gain1 : Gain  Gain=com_c
  Sum2 : Sum  Inputs=|+-
  Sum3 : Sum  Inputs=|++
  Transfer Fcn3 : TransferFcn  Numerator=a_c  Denominator=[1 a_c]
  Unit Delay1 : UnitDelay  SampleTime=-1
  Zero-Order Hold3 : ZeroOrderHold  SampleTime=-1
  inv1 : Saturate  UpperLimit=p_limits(1)  LowerLimit=-p_limits(1)
  Out1 : Outport
  wires:
  Transfer Fcn3/1 -> inv1/1
  Gain1/1 -> Sum3/1
  inv1/1 -> Unit Delay1/1, Out1/1
  In1/1 -> Sum2/1
  Unit Delay1/1 -> Sum2/2, Sum3/2
  Sum2/1 -> Gain1/1
  Zero-Order Hold3/1 -> Transfer Fcn3/1
  Sum3/1 -> Zero-Order Hold3/1

== system twin/Subsystem3/first orde7 ==
  In1 : Inport
  Gain1 : Gain  Gain=com_c
  Sum2 : Sum  Inputs=|+-
  Sum3 : Sum  Inputs=|++
  Transfer Fcn3 : TransferFcn  Numerator=a_c  Denominator=[1 a_c]
  Unit Delay1 : UnitDelay  SampleTime=-1
  Zero-Order Hold3 : ZeroOrderHold  SampleTime=-1
  inv1 : Saturate  UpperLimit=p_limits(1)  LowerLimit=-p_limits(1)
  Out1 : Outport
  wires:
  Transfer Fcn3/1 -> inv1/1
  Gain1/1 -> Sum3/1
  inv1/1 -> Unit Delay1/1, Out1/1
  In1/1 -> Sum2/1
  Unit Delay1/1 -> Sum2/2, Sum3/2
  Sum2/1 -> Gain1/1
  Zero-Order Hold3/1 -> Transfer Fcn3/1
  Sum3/1 -> Zero-Order Hold3/1

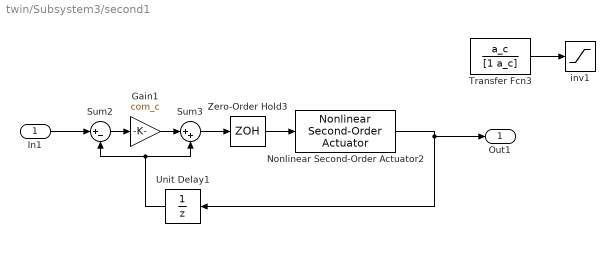
== system twin/Subsystem3/second1 ==
  In1 : Inport
  Gain1 : Gain  Gain=com_c
  Nonlinear Second-Order Actuator2 : aerolibactuator/Nonlinear Second-Order Actuator  wn_fin=200  z_fin=0.7  fin_max=(p_limits(1))*pi/180  fin_min=(-p_limits(1))*pi/180  fin_maxrate=v_limits(1)*pi/180  fin_act_0=0  fin_act_vel=0
      settings: SourceProductName=Aerospace Blockset  SourceProductBaseCode=AE
  Sum2 : Sum  Inputs=|+-
  Sum3 : Sum  Inputs=|++
  Transfer Fcn3 : TransferFcn  Numerator=a_c  Denominator=[1 a_c]
  Unit Delay1 : UnitDelay  SampleTime=-1
  Zero-Order Hold3 : ZeroOrderHold  SampleTime=-1
  inv1 : Saturate  UpperLimit=p_limits(1)  LowerLimit=-p_limits(1)
  Out1 : Outport
  wires:
  Gain1/1 -> Sum3/1
  Nonlinear Second-Order Actuator2/1 -> Unit Delay1/1, Out1/1
  In1/1 -> Sum2/1
  Unit Delay1/1 -> Sum2/2, Sum3/2
  Sum2/1 -> Gain1/1
  Sum3/1 -> Zero-Order Hold3/1
  ? -> Transfer Fcn3/1
  Transfer Fcn3/1 -> inv1/1
  Zero-Order Hold3/1 -> Nonlinear Second-Order Actuator2/1

== system twin/Subsystem4/Subsystem1 ==
  In1 : Inport
  Transfer Fcn3 : TransferFcn  Numerator=a_c  Denominator=[1 a_c]
  Zero-Order Hold3 : ZeroOrderHold  SampleTime=-1
  inv1 : Saturate  UpperLimit=p_limits(1)  LowerLimit=-p_limits(1)
  Out1 : Outport
  wires:
  Transfer Fcn3/1 -> inv1/1
  inv1/1 -> Out1/1
  Zero-Order Hold3/1 -> Transfer Fcn3/1
  In1/1 -> Zero-Order Hold3/1

== system twin/Subsystem4/Subsystem2 ==
  In1 : Inport
  Transfer Fcn3 : TransferFcn  Numerator=a_c  Denominator=[1 a_c]
  Zero-Order Hold3 : ZeroOrderHold  SampleTime=-1
  inv1 : Saturate  UpperLimit=p_limits(1)  LowerLimit=-p_limits(1)
  Out1 : Outport
  wires:
  Transfer Fcn3/1 -> inv1/1
  inv1/1 -> Out1/1
  Zero-Order Hold3/1 -> Transfer Fcn3/1
  In1/1 -> Zero-Order Hold3/1

== system twin/Subsystem4/Subsystem3 ==
  In1 : Inport
  Transfer Fcn3 : TransferFcn  Numerator=a_c  Denominator=[1 a_c]
  Zero-Order Hold3 : ZeroOrderHold  SampleTime=-1
  inv1 : Saturate  UpperLimit=p_limits(1)  LowerLimit=-p_limits(1)
  Out1 : Outport
  wires:
  Transfer Fcn3/1 -> inv1/1
  inv1/1 -> Out1/1
  Zero-Order Hold3/1 -> Transfer Fcn3/1
  In1/1 -> Zero-Order Hold3/1

== system twin/Subsystem4/Subsystem4 ==
  In1 : Inport
  Transfer Fcn3 : TransferFcn  Numerator=a_c  Denominator=[1 a_c]
  Zero-Order Hold3 : ZeroOrderHold  SampleTime=-1
  inv1 : Saturate  UpperLimit=p_limits(1)  LowerLimit=-p_limits(1)
  Out1 : Outport
  wires:
  Transfer Fcn3/1 -> inv1/1
  inv1/1 -> Out1/1
  Zero-Order Hold3/1 -> Transfer Fcn3/1
  In1/1 -> Zero-Order Hold3/1

== system twin/Subsystem4/Subsystem6 ==
  In1 : Inport
  Transfer Fcn3 : TransferFcn  Numerator=a_c  Denominator=[1 a_c]
  Zero-Order Hold3 : ZeroOrderHold  SampleTime=-1
  inv1 : Saturate  UpperLimit=p_limits(1)  LowerLimit=-p_limits(1)
  Out1 : Outport
  wires:
  Transfer Fcn3/1 -> inv1/1
  inv1/1 -> Out1/1
  Zero-Order Hold3/1 -> Transfer Fcn3/1
  In1/1 -> Zero-Order Hold3/1

== system twin/Subsystem4/Subsystem7 ==
  In1 : Inport
  Transfer Fcn3 : TransferFcn  Numerator=a_c  Denominator=[1 a_c]
  Zero-Order Hold3 : ZeroOrderHold  SampleTime=-1
  inv1 : Saturate  UpperLimit=p_limits(1)  LowerLimit=-p_limits(1)
  Out1 : Outport
  wires:
  Transfer Fcn3/1 -> inv1/1
  inv1/1 -> Out1/1
  Zero-Order Hold3/1 -> Transfer Fcn3/1
  In1/1 -> Zero-Order Hold3/1

== system twin/Subsystem4/Subsystem8 ==
  In1 : Inport
  Transfer Fcn3 : TransferFcn  Numerator=a_c  Denominator=[1 a_c]
  Zero-Order Hold3 : ZeroOrderHold  SampleTime=-1
  inv1 : Saturate  UpperLimit=p_limits(1)  LowerLimit=-p_limits(1)
  Out1 : Outport
  wires:
  Transfer Fcn3/1 -> inv1/1
  inv1/1 -> Out1/1
  Zero-Order Hold3/1 -> Transfer Fcn3/1
  In1/1 -> Zero-Order Hold3/1

== system twin/Subsystem4/Subsystem9 ==
  In1 : Inport
  To Workspace1 : ToWorkspace  VariableName=wls_c_out_off  SaveFormat=Timeseries  SampleTime=-1
  To Workspace2 : ToWorkspace  VariableName=wls_c_in_off  SaveFormat=Timeseries  SampleTime=-1
  Transfer Fcn3 : TransferFcn  Numerator=a_c  Denominator=[1 a_c]
  Zero-Order Hold3 : ZeroOrderHold  SampleTime=-1
  inv1 : Saturate  UpperLimit=p_limits(1)  LowerLimit=-p_limits(1)
  Out1 : Outport
  wires:
  Transfer Fcn3/1 -> inv1/1
  Zero-Order Hold3/1 -> Transfer Fcn3/1
  In1/1 -> Zero-Order Hold3/1, To Workspace2/1
  inv1/1 -> To Workspace1/1, Out1/1
